simulink model "sat"  (R2017a)
settings: Solver=VariableStepAuto  StartTime=0.0  StopTime=25  RelTol=1e-3
settings Model: Creator=HP  LastModifiedBy=HP

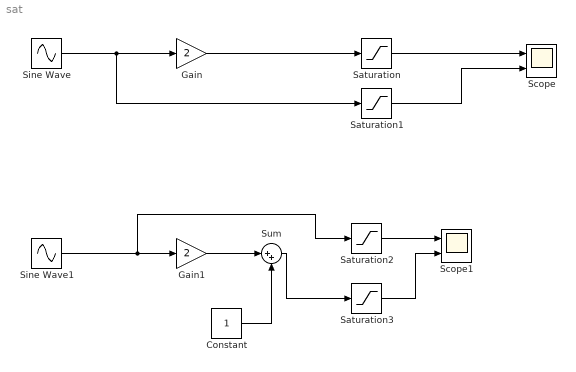
== system sat ==
  Constant : Constant
  Gain : Gain  Gain=2
  Gain1 : Gain  Gain=2
  Saturation{,1..3} (4 alike) : Saturate  UpperLimit=1  LowerLimit=-1
  Scope : Scope  NumInputPorts=2
  Scope1 : Scope  NumInputPorts=2
  Sine Wave : Sin  SampleTime=0
  Sine Wave1 : Sin  SampleTime=0
  Sum : Sum  Inputs=|++
  wires:
  Sine Wave/1 -> Gain/1, Saturation1/1
  Gain/1 -> Saturation/1
  Sum/1 -> Saturation3/1
  Gain1/1 -> Sum/1
  Sine Wave1/1 -> Saturation2/1, Gain1/1
  Constant/1 -> Sum/2
  Saturation/1 -> Scope/1
  Saturation1/1 -> Scope/2
  Saturation2/1 -> Scope1/1
  Saturation3/1 -> Scope1/2
